simulink model "temp_test"  (R2022a)
settings: Solver=VariableStepAuto  StartTime=0.0  StopTime=10000  RelTol=1e-3
values from neighbouring files (symbols this model uses):
  Ts = 2    [chamber_params.m]    (also in system_ident.m = 1)
undefined symbols (not defined in the file or in its folder): room
libraries: fl_lib x13, nesl_utility x6
settings Model: Creator=mmarq  LastModifiedBy=mmarq

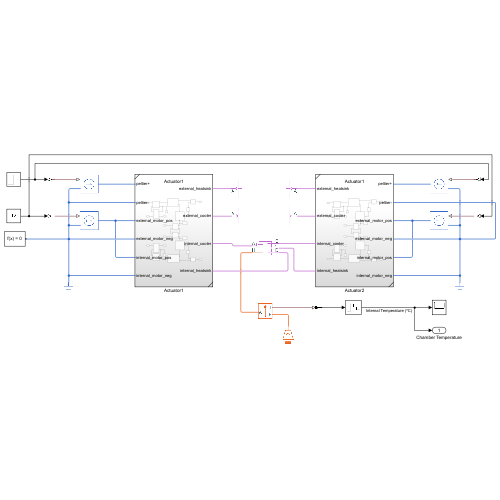
[thumbnail: Simulink's stored preview of the top-level diagram]
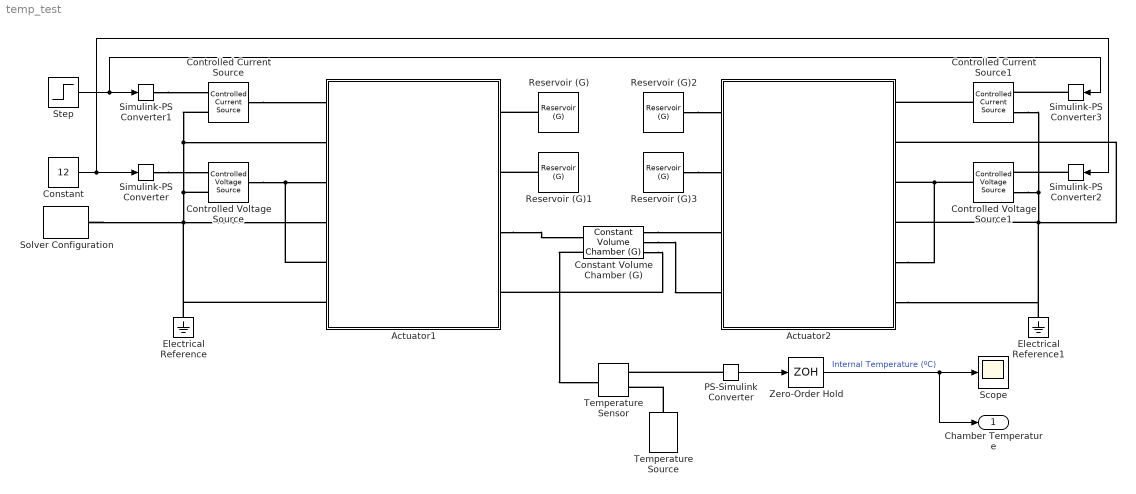
== system temp_test ==
  Actuator1 : Subsystem  ReferencedSubsystem=Actuator1
      settings: PortSchema="{\"entries\":[{\"content\":{\"sides\":[{\"content\":{\"connectorIds\":[\"LConn1\",\"LConn2\",\"LConn3\",\"LConn4\",\"LConn7\",\"LConn8\"]},\"type\":\"ConnectorPlacement.EquallySpacedRectSide\",\"uuid\":\"d457bfca-5b88-4301-b763-1a1ef357e8f7\"},{\"content\":{\"connectorIds\":[\"LConn5\",\"LConn6\",\"LConn9\",\"LConn10\"],\"side\":\"RIGHT\"},\"type\":\"ConnectorPlacement.EquallySpacedRectSide\",\"uuid\":\"6d21a9da-5af6-404c-9aaa-5fa645f96412\"},{\"content\":{\"connectorIds\":[],\"side\":\"TOP\"},\"type\":\"ConnectorPlacement.EquallySpacedRectSide\",\"uuid\":\"c6c34e02-cd8b-4639-9d69-df950db50ed6\"},{\"content\":{\"connectorIds\":[],\"side\":\"BOTTOM\"},\"type\":\"ConnectorPlacement.EquallySpacedRectSide\",\"uuid\":\"2eb52547-80cf-413a-b1f5-6d0ef02648c5\"}]},\"type\":\"ConnectorPlacement.EquallySpacedConnector\",\"uuid\":\"bd541323-b134-4609-9d7e-6e951cab5180\"}],\"packageUris\":[\"http://schema.mathworks.com/mf0/Connector/R2020b\"],\"version\":\"1.0\"}"
  Actuator2 : Subsystem  ReferencedSubsystem=Actuator1
      settings: PortSchema="{\"entries\":[{\"content\":{\"sides\":[{\"content\":{\"connectorIds\":[\"LConn1\",\"LConn2\",\"LConn3\",\"LConn4\",\"LConn7\",\"LConn8\"]},\"type\":\"ConnectorPlacement.EquallySpacedRectSide\",\"uuid\":\"d457bfca-5b88-4301-b763-1a1ef357e8f7\"},{\"content\":{\"connectorIds\":[\"LConn5\",\"LConn6\",\"LConn9\",\"LConn10\"],\"side\":\"RIGHT\"},\"type\":\"ConnectorPlacement.EquallySpacedRectSide\",\"uuid\":\"6d21a9da-5af6-404c-9aaa-5fa645f96412\"},{\"content\":{\"connectorIds\":[],\"side\":\"TOP\"},\"type\":\"ConnectorPlacement.EquallySpacedRectSide\",\"uuid\":\"c6c34e02-cd8b-4639-9d69-df950db50ed6\"},{\"content\":{\"connectorIds\":[],\"side\":\"BOTTOM\"},\"type\":\"ConnectorPlacement.EquallySpacedRectSide\",\"uuid\":\"2eb52547-80cf-413a-b1f5-6d0ef02648c5\"}]},\"type\":\"ConnectorPlacement.EquallySpacedConnector\",\"uuid\":\"bd541323-b134-4609-9d7e-6e951cab5180\"}],\"packageUris\":[\"http://schema.mathworks.com/mf0/Connector/R2020b\"],\"version\":\"1.0\"}"
  Constant : Constant  Value=12
  Constant Volume Chamber (G) : fl_lib/Gas/Elements/Constant Volume Chamber (G)  volume=0.000288 m^3  num_ports=foundation.enum.num_ports.four  area_A=0.0016 m^2  area_B=0.0016 m^2  area_C=0.0004 m^2  area_D=0.0004 m^2  p_I_specify=off  p_I_priority=High  p_I=0.101325 MPa  p_I_nominal_specify=off  p_I_nominal_unit=MPa  p_I_nominal_value=1  T_I_specify=on  T_I_priority=High  T_I=room.env_temp + 273 K  T_I_nominal_specify=off  T_I_nominal_unit=K  T_I_nominal_value=1  rho_chamber_specify=off  rho_chamber_priority=None  rho_chamber=1.2 kg/m^3  rho_chamber_nominal_specify=off  rho_chamber_nominal_unit=kg/m^3  rho_chamber_nominal_value=1
      settings: SourceProductBaseCode=PW,SS,VE  InternalSimscapePortConfiguration="{\"Bottom\":[],\"Left\":[{\"id\":\"A\",\"label\":\"A\",\"type\":\"foundation.gas.gas\"},{\"id\":\"H\",\"label\":\"H\",\"type\":\"foundation.thermal.thermal\"}],\"Right\":[{\"id\":\"B\",\"label\":\"B\",\"type\":\"foundation.gas.gas\"},{\"id\":\"C\",\"label\":\"C\",\"type\":\"foundation.gas.gas\"},{\"id\":\"D\",\"label\":\"D\",\"type\":\"foundation.gas.gas\"}],\"Top\":[]}"
  Controlled Current Source : fl_lib/Electrical/Electrical Sources/Controlled Current Source
      settings: SourceProductBaseCode=PW,SS,VE
  Controlled Current Source1 : fl_lib/Electrical/Electrical Sources/Controlled Current Source
      settings: SourceProductBaseCode=PW,SS,VE
  Controlled Voltage Source : fl_lib/Electrical/Electrical Sources/Controlled Voltage Source
      settings: SourceProductBaseCode=PW,SS,VE
  Controlled Voltage Source1 : fl_lib/Electrical/Electrical Sources/Controlled Voltage Source
      settings: SourceProductBaseCode=PW,SS,VE
  Electrical Reference : fl_lib/Electrical/Electrical Elements/Electrical Reference
      settings: SourceProductBaseCode=PW,SS,VE
  Electrical Reference1 : fl_lib/Electrical/Electrical Elements/Electrical Reference
      settings: SourceProductBaseCode=PW,SS,VE
  PS-Simulink Converter : nesl_utility/PS-Simulink Converter  PhysicalDomain=network_engine_domain  SubClassName=ps_output  LeftPortType=input  RightPortType=output  PseudoPeriodic=off  Frequencies=[]  VectorFormat=1-D array  Unit=inherit  AffineConversion=off
      settings: SourceProductBaseCode=SS,PW,VE
  Reservoir (G){,1..3} (4 alike) : fl_lib/Gas/Elements/Reservoir (G)  pressure_spec=foundation.enum.pressure_spec.atmospheric  reservoir_pressure=0.101325 MPa  reservoir_temperature=room.env_temp + 273 K  area_A=0.01 m^2
      settings: SourceProductBaseCode=PW,SS,VE
  Scope : Scope
  Simulink-PS Converter{,1..3} (4 alike) : nesl_utility/Simulink-PS Converter  PhysicalDomain=network_engine_domain  SubClassName=ps_input  LeftPortType=input  RightPortType=output  PseudoPeriodic=off  Frequencies=[]  NoiseDistribution=none  NoiseParameters=[]  Unit=1  AffineConversion=off  FilteringAndDerivatives=provide  SimscapeFilterOrder=1  InputFilterTimeConstant=0.001  UdotUserProvided=0
      settings: SourceProductBaseCode=SS,PW,VE
  Solver Configuration : nesl_utility/Solver Configuration  PhysicalDomain=network_engine_domain  SubClassName=solver  LeftPortType=input  RightPortType=generic  Tones=[]  Harmonics=[]  SimulateNoise=off  Profile=off  UseLocalSampling=off  EnableSwitchedLinearOptims=on  FrequencyDomain=off  UseCCode=off  RelTol=0.001  AbsTol=0.001  MinStep=1e-09  ToWorkspace=off  RevertToSquareIcSolve=off  NumHomotopyIterations=100  PhasorMode=off  PhasorModeNumHarmonics=1  IndexReductionMethod=DerivativeReplacement  DoDC=off  ResidualTolerance=1e-09  UseLocalSolver=off  LocalSolverChoice=NE_BACKWARD_EULER_ADVANCER  LocalSolverSampleTime=0.001  DoFixedCost=off  MaxNonlinIter=3  MaxModeIter=2  ComputeImpulses=off  ImpulseIterations=2  LinearAlgebra=auto  LinearAlgebraNumThread=0  EquationFormulation=NE_TIME_EF  DelaysMemoryBudget=1024  AutomaticFiltering=on  FilteringTimeConstant=0.001  PartitionStorageMethod=AS_NEEDED  PartitionMemoryBudget=1024  PartitionMethod=ROBUST
      settings: SourceProductBaseCode=SS,PW,VE
  Step : Step  Time=0  SampleTime=0
  Temperature Sensor : fl_lib/Thermal/Thermal Sensors/Temperature Sensor
      settings: SourceProductBaseCode=PW,SS,VE
  Temperature Source : fl_lib/Thermal/Thermal Sources/Temperature Source  temperature=273 K
      settings: SourceProductBaseCode=PW,SS,VE
  Zero-Order Hold : ZeroOrderHold  SampleTime=Ts
  Chamber Temperature : Outport
  wires:
  Constant/1 -> Simulink-PS Converter/1, Simulink-PS Converter2/1
  Step/1 -> Simulink-PS Converter3/1, Simulink-PS Converter1/1
  PS-Simulink Converter/1 -> Zero-Order Hold/1
  Zero-Order Hold/1 -> Chamber Temperature/1, Scope/1  "Internal Temperature (ºC)"
  connections:
  Reservoir (G)/LConn1 -- Actuator1/LConn5
  Reservoir (G)1/LConn1 -- Actuator1/LConn6
  Controlled Current Source/LConn1 -- Actuator1/LConn1
  Controlled Voltage Source/LConn1 -- Actuator1/LConn7 -- Actuator1/LConn3
  Controlled Current Source/RConn2 -- Actuator1/LConn2 -- Controlled Voltage Source/RConn2 -- Actuator1/LConn8 -- Electrical Reference/LConn1 -- Actuator1/LConn4 -- Solver Configuration/RConn1
  Simulink-PS Converter/RConn1 -- Controlled Voltage Source/RConn1
  Simulink-PS Converter1/RConn1 -- Controlled Current Source/RConn1
  Controlled Current Source1/RConn2 -- Controlled Voltage Source1/RConn2 -- Actuator2/LConn2 -- Electrical Reference1/LConn1 -- Actuator2/LConn8 -- Actuator2/LConn4
  Controlled Voltage Source1/LConn1 -- Actuator2/LConn3 -- Actuator2/LConn7
  Reservoir (G)3/LConn1 -- Actuator2/LConn6
  Simulink-PS Converter3/RConn1 -- Controlled Current Source1/RConn1
  Controlled Current Source1/LConn1 -- Actuator2/LConn1
  Simulink-PS Converter2/RConn1 -- Controlled Voltage Source1/RConn1
  Reservoir (G)2/LConn1 -- Actuator2/LConn5
  Actuator1/LConn9 -- Constant Volume Chamber (G)/LConn1
  Constant Volume Chamber (G)/RConn1 -- Actuator2/LConn9
  Constant Volume Chamber (G)/RConn2 -- Actuator2/LConn10
  Constant Volume Chamber (G)/RConn3 -- Actuator1/LConn10
  Constant Volume Chamber (G)/LConn2 -- Temperature Sensor/LConn1
  Temperature Source/LConn1 -- Temperature Sensor/RConn1
  PS-Simulink Converter/LConn1 -- Temperature Sensor/RConn2
